simulink model "fuelCycle_w_trapping"  (R2023b)
settings: Solver=ode15s  StartTime=0.0  StopTime=sim_time  MinStep=1e-4  RelTol=1e-4
values from neighbouring files (symbols this model uses):
  AF = 0.90    (= 0.9)    [FC_scenario_inputData.m]    (also in inputData.m = 70)
  eta2 = 0.95    [FC_scenario_inputData.m]    (also in inputData.m)
  f51 = 0.33    [FC_scenario_inputData.m]    (also in inputData.m)
  f53 = 0.33    [FC_scenario_inputData.m]    (also in inputData.m)
  f54 = 1 - f51 - f53 - f56    (= 0.3399)    [FC_scenario_inputData.m]    (also in inputData.m)
  f96 = 0.1    [FC_scenario_inputData.m]    (also in inputData.m)
  f_dir = 0.7    [FC_scenario_inputData.m]    (also in inputData.m = 0.3)
  fp3 = 1e-4    (= 0.0001)    [FC_scenario_inputData.m]    (also in inputData.m; parametric_analysis_f_p_trap.m = f_p(i))
  fp4 = 1e-4    (= 0.0001)    [FC_scenario_inputData.m]    (also in inputData.m; parametric_analysis_f_p_trap.m = f_p(i))
  I_s_0 = 1.85    [fuelCycleSimulator.m]    (also in parametric_analysis_f_p_trap.m = 0.8; utilities.m = I_s_0 - abs(margin) + inventory_accuracy)
  lambda = 1.73e-9    (= 1.73e-09)    [FC_scenario_inputData.m]    (also in inputData.m)
  N_dot = 9.3e-7    (= 9.3e-07)    [FC_scenario_inputData.m]    (also in inputData.m)
  n_trap_structural = n_trap_vcrti    (= 0.0001)    [inputData_trapping.m]    (also in parametric_analysis_trapping.m = n_trap_array(j))
  n_trap_tungsten_intrinsic = 3.5e-4    (= 0.00035)    [inputData_trapping.m]
  T1 = 1/((1 + epsi)/tau1 + lambda)    [FC_scenario_inputData.m]    (also in inputData.m)
  T12 = 1/((1 + epsi)/tau12 + lambda)    [FC_scenario_inputData.m]    (also in inputData.m)
  T2 = 1/((1 + epsi)/tau2 + lambda)    [FC_scenario_inputData.m]    (also in inputData.m)
  T3 = 1/((1 + 0)/tau3 + lambda)    [FC_scenario_inputData.m]    (also in inputData.m)
  T4 = 1/((1 + 0)/tau4 + lambda)    [FC_scenario_inputData.m]    (also in inputData.m)
  T7 = 1/((1 + epsi)/tau7 + lambda)    [FC_scenario_inputData.m]    (also in inputData.m)
  T8 = 1/((1 + epsi)/tau8 + lambda)    [FC_scenario_inputData.m]    (also in inputData.m)
  T9 = 1/((1 + epsi)/tau9 + lambda)    [FC_scenario_inputData.m]    (also in inputData.m)
  T_replacement = 1.7*8760*3600    (= 53611200)    [inputData.m]
  tau1 = 1.25*3600    (= 4500)    [FC_scenario_inputData.m]    (also in inputData.m)
  tau12 = 100    [FC_scenario_inputData.m]    (also in inputData.m)
  tau2 = 1*24*3600    (= 86400)    [FC_scenario_inputData.m]    (also in inputData.m)
  tau3 = 1000    [FC_scenario_inputData.m]    (also in inputData.m)
  tau4 = 1000    [FC_scenario_inputData.m]    (also in inputData.m)
  tau5 = 1000    [FC_scenario_inputData.m]    (also in inputData.m)
  tau6 = 3600    [FC_scenario_inputData.m]    (also in inputData.m)
  tau7 = 600    [FC_scenario_inputData.m]    (also in inputData.m)
  tau8 = 0.1*3600    (= 360)    [FC_scenario_inputData.m]    (also in inputData.m = 3600)
  tau9 = 0.9*3600    (= 3240)    [FC_scenario_inputData.m]    (also in inputData.m = 10800)
  tau_detrap_structural = 1 / nu_detrap_structural* relaxation_coefficient    [inputData_trapping.m]
  TBE = 0.02    [FC_scenario_inputData.m]    (also in inputData.m; parametric_analysis_f_p_trap.m = TBE_array(j); parametric_analysis_trapping.m)
  TBR = 1.096    [fuelCycleSimulator.m]    (also in parametric_analysis_f_p_trap.m = 1.048; parametric_analysis_trapping.m = 1.06; utilities.m = TBR_start)
libraries: arc x5
settings Model: SimulationMode=accelerator  Creator=smesc  LastModifiedBy=smesc
settings SolverCC: InitialStep=1e-4  MaxConsecutiveMinStep=10  ShapePreserveControl=EnableAll  ZeroCrossAlgorithm=Adaptive
settings OptimizationCC: ReuseModelBlockBuffer=off
settings ModelReferenceCC: EnableRefExpFcnMdlSchedulingChecks=on

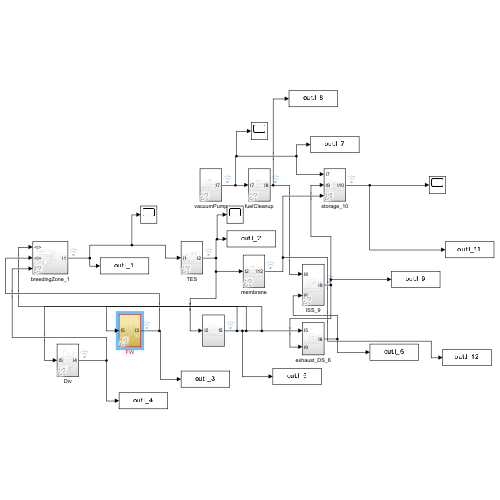
[thumbnail: Simulink's stored preview of the top-level diagram]
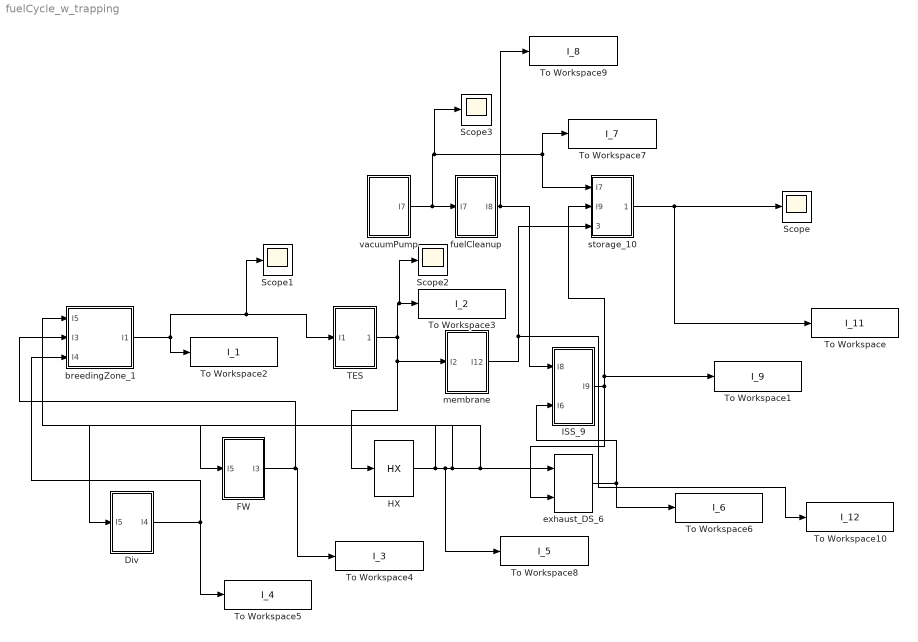
== system fuelCycle_w_trapping ==
  Div : Subsystem  AncestorBlock=arc/divertor_4
      settings: LibrarySourceBlock=arc/divertor_4
  FW : Subsystem  AncestorBlock=arc/FW_3
      settings: LibrarySourceBlock=arc/FW_3
  HX : arc/HX  Tag=HX  SystemSampleTime=-1  VariantActivationTime=update diagram  AllowFlexibleInterface=on  Latency=0  AutoFrameSizeCalculation=off
  ISS_9 : Subsystem  AncestorBlock=arc/ISS_9
      settings: LibrarySourceBlock=arc/ISS_9
  Scope{,1..3} (4 alike) : Scope
  TES : Subsystem  AncestorBlock=arc/TES_2
      settings: LibrarySourceBlock=arc/TES_2
  To Workspace : ToWorkspace  VariableName=I_11  SampleTime=-1
  To Workspace1 : ToWorkspace  VariableName=I_9  SampleTime=-1
  To Workspace10 : ToWorkspace  VariableName=I_12  SampleTime=-1
  To Workspace2 : ToWorkspace  VariableName=I_1  SampleTime=-1
  To Workspace3 : ToWorkspace  VariableName=I_2  SampleTime=-1
  To Workspace4 : ToWorkspace  VariableName=I_3  SampleTime=-1
  To Workspace5 : ToWorkspace  VariableName=I_4  SampleTime=-1
  To Workspace6 : ToWorkspace  VariableName=I_6  SampleTime=-1
  To Workspace7 : ToWorkspace  VariableName=I_7  SampleTime=-1
  To Workspace8 : ToWorkspace  VariableName=I_5  SampleTime=-1
  To Workspace9 : ToWorkspace  VariableName=I_8  SampleTime=-1
  breedingZone_1 : Subsystem  AncestorBlock=arc/breedingZone_1
      settings: LibrarySourceBlock=arc/breedingZone_1
  exhaust_DS_6 : arc/exhaust_DS  SystemSampleTime=-1  VariantActivationTime=update diagram  AllowFlexibleInterface=on  Latency=0  AutoFrameSizeCalculation=off
      link override Gain: Gain=f56/tau5
  fuelCleanup : Subsystem  AncestorBlock=arc/fuelCleanUp
  membrane : Subsystem  AncestorBlock=arc/fuelCleanUp_8
      settings: LibrarySourceBlock=arc/fuelCleanUp_8
  storage_10 : Subsystem  AncestorBlock=arc/storage_10
      settings: LibrarySourceBlock=arc/storage_10
  vacuumPump : Subsystem  AncestorBlock=arc/pump_7
      settings: LibrarySourceBlock=arc/pump_7
  wires:
  breedingZone_1/1(I1) -> Scope1/1, TES/1(I1), To Workspace2/1
  storage_10/1(I10) -> To Workspace/1, Scope/1
  FW/1(I3) -> breedingZone_1/2(I3), To Workspace4/1
  Div/1(I4) -> breedingZone_1/3(I4), To Workspace5/1
  membrane/1(I12) -> To Workspace10/1, storage_10/3(I12)
  fuelCleanup/1(I8) -> To Workspace9/1, ISS_9/1(I8)
  vacuumPump/1(I7) -> Scope3/1, To Workspace7/1, storage_10/1(I7), fuelCleanup/1(I7)
  exhaust_DS_6/1 -> ISS_9/2(I6), To Workspace6/1
  ISS_9/1(I9) -> exhaust_DS_6/2, storage_10/2(I9), To Workspace1/1
  HX/1 -> FW/1(I5), To Workspace8/1, Div/1(I5), exhaust_DS_6/1, breedingZone_1/1(I5)
  TES/1(Output) -> Scope2/1, To Workspace3/1, membrane/1(I2), HX/1

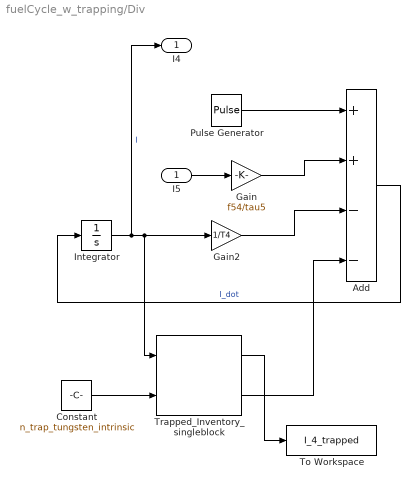
== system fuelCycle_w_trapping/Div ==
  I5 : Inport
  Add : Sum  Inputs=++--
  Constant : Constant  Value=n_trap_tungsten_intrinsic
  Gain : Gain  Gain=f54/tau5
  Gain2 : Gain  Gain=1/T4
  Integrator : Integrator
  Pulse Generator : DiscretePulseGenerator  PulseType=Time based  Amplitude=fp4*N_dot/TBE  Period=1800  PulseWidth=AF
  To Workspace : ToWorkspace  VariableName=I_4_trapped  SampleTime=-1
  Trapped_Inventory_singleblock : arc/Trapped_Inventory_singleblock  SystemSampleTime=-1  VariantActivationTime=update diagram  AllowFlexibleInterface=on  Latency=0  AutoFrameSizeCalculation=off
      link override Trap_detrap_ml2: tau_detrap=tau_detrap_tungsten(1)  n_solute=n_solute_tungsten  PM_host=PM_tungsten  M_host=PM_tungsten  tau_trap=tau_trap_tungsten
  I4 : Outport
  wires:
  Pulse Generator/1 -> Add/1
  Gain/1 -> Add/2
  Integrator/1 -> Trapped_Inventory_singleblock/1, Gain2/1, I4/1  "I"
  Add/1 -> Integrator/1  "I_dot"
  Gain2/1 -> Add/3
  I5/1 -> Gain/1
  Trapped_Inventory_singleblock/1 -> To Workspace/1
  Trapped_Inventory_singleblock/2 -> Add/4
  Constant/1 -> Trapped_Inventory_singleblock/2

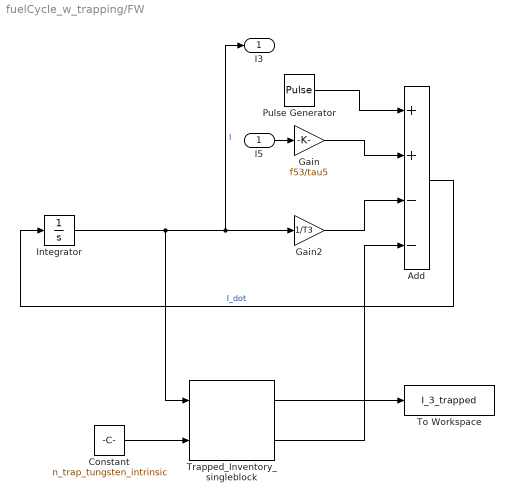
== system fuelCycle_w_trapping/FW ==
  I5 : Inport
  Add : Sum  Inputs=++--
  Constant : Constant  Value=n_trap_tungsten_intrinsic
  Gain : Gain  Gain=f53/tau5
  Gain2 : Gain  Gain=1/T3
  Integrator : Integrator
  Pulse Generator : DiscretePulseGenerator  PulseType=Time based  Amplitude=fp3*N_dot/TBE  Period=1800  PulseWidth=AF
  To Workspace : ToWorkspace  VariableName=I_3_trapped  SampleTime=-1
  Trapped_Inventory_singleblock : arc/Trapped_Inventory_singleblock  SystemSampleTime=-1  VariantActivationTime=update diagram  AllowFlexibleInterface=on  Latency=0  AutoFrameSizeCalculation=off
      link override Trap_detrap_ml2: tau_detrap=tau_detrap_tungsten(1)  n_solute=n_solute_tungsten  PM_host=PM_tungsten  M_host=M_tungsten  tau_trap=tau_trap_tungsten
  I3 : Outport
  wires:
  Gain2/1 -> Add/3
  Pulse Generator/1 -> Add/1
  Integrator/1 -> Gain2/1, I3/1, Trapped_Inventory_singleblock/1  "I"
  Add/1 -> Integrator/1  "I_dot"
  Gain/1 -> Add/2
  I5/1 -> Gain/1
  Trapped_Inventory_singleblock/2 -> Add/4
  Trapped_Inventory_singleblock/1 -> To Workspace/1
  Constant/1 -> Trapped_Inventory_singleblock/2

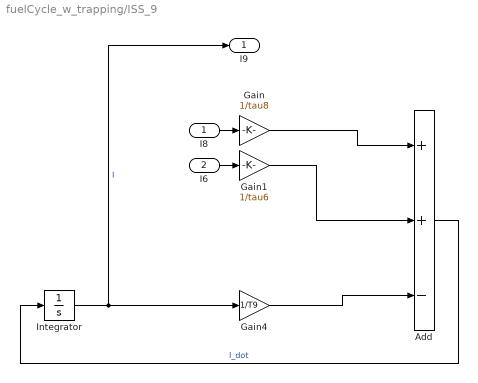
== system fuelCycle_w_trapping/ISS_9 ==
  I8 : Inport
  I6 : Inport  Port=2
  Add : Sum  Inputs=++-
  Gain : Gain  Gain=1/tau8
  Gain1 : Gain  Gain=1/tau6
  Gain4 : Gain  Gain=1/T9
  Integrator : Integrator
  I9 : Outport
  wires:
  I8/1 -> Gain/1
  Gain1/1 -> Add/2
  I6/1 -> Gain1/1
  Add/1 -> Integrator/1  "I_dot"
  Integrator/1 -> Gain4/1, I9/1  "I"
  Gain/1 -> Add/1
  Gain4/1 -> Add/3

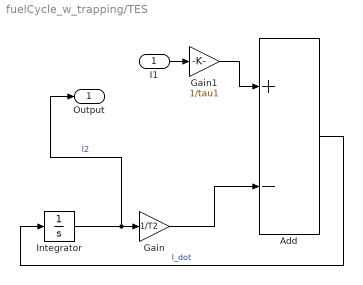
== system fuelCycle_w_trapping/TES ==
  I1 : Inport
  Add : Sum  Inputs=+-
  Gain : Gain  Gain=1/T2
  Gain1 : Gain  Gain=1/tau1
  Integrator : Integrator
  Output : Outport
  wires:
  Gain/1 -> Add/2
  I1/1 -> Gain1/1
  Gain1/1 -> Add/1
  Integrator/1 -> Gain/1, Output/1  "I2"
  Add/1 -> Integrator/1  "I_dot"

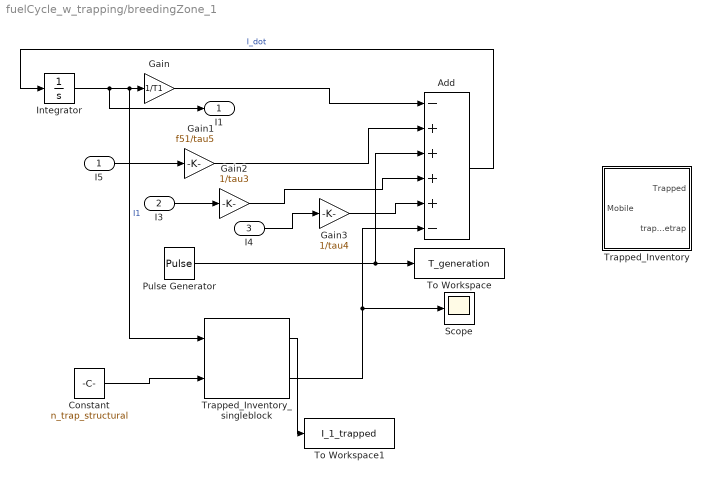
== system fuelCycle_w_trapping/breedingZone_1 ==
  I5 : Inport
  I3 : Inport  Port=2
  I4 : Inport  Port=3
  Add : Sum  Inputs=-++++-
  Constant : Constant  Value=n_trap_structural
  Gain : Gain  Gain=1/T1
  Gain1 : Gain  Gain=f51/tau5
  Gain2 : Gain  Gain=1/tau3
  Gain3 : Gain  Gain=1/tau4
  Integrator : Integrator
  Pulse Generator : DiscretePulseGenerator  PulseType=Time based  Amplitude=N_dot * TBR  Period=1800  PulseWidth=AF
  Scope : Scope
  To Workspace : ToWorkspace  VariableName=T_generation  SaveFormat=Timeseries  SampleTime=-1
  To Workspace1 : ToWorkspace  VariableName=I_1_trapped  SampleTime=-1
  Trapped_Inventory : Subsystem  AncestorBlock=arc/Trapped_Inventory
  Trapped_Inventory_singleblock : arc/Trapped_Inventory_singleblock  SystemSampleTime=-1  VariantActivationTime=update diagram  AllowFlexibleInterface=on  Latency=0  AutoFrameSizeCalculation=off
      link override Trap_detrap_ml2: tau_detrap=tau_detrap_structural  n_solute=n_solute_structural
  I1 : Outport
  wires:
  Add/1 -> Integrator/1  "I_dot"
  Gain1/1 -> Add/2
  Integrator/1 -> Trapped_Inventory_singleblock/1, Gain/1, I1/1  "I1"
  Gain/1 -> Add/1
  I5/1 -> Gain1/1
  Pulse Generator/1 -> Add/3, To Workspace/1
  I3/1 -> Gain2/1
  Gain2/1 -> Add/4
  I4/1 -> Gain3/1
  Gain3/1 -> Add/5
  Constant/1 -> Trapped_Inventory_singleblock/2
  Trapped_Inventory_singleblock/1 -> To Workspace1/1
  Trapped_Inventory_singleblock/2 -> Add/6, Scope/1

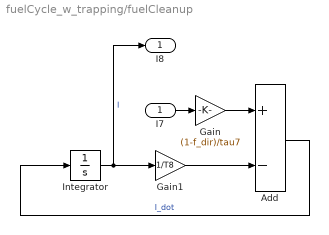
== system fuelCycle_w_trapping/fuelCleanup ==
  I7 : Inport
  Add : Sum  Inputs=+-
  Gain : Gain  Gain=(1-f_dir)/tau7
  Gain1 : Gain  Gain=1/T8
  Integrator : Integrator
  I8 : Outport
  wires:
  I7/1 -> Gain/1
  Gain1/1 -> Add/2
  Add/1 -> Integrator/1  "I_dot"
  Integrator/1 -> Gain1/1, I8/1  "I"
  Gain/1 -> Add/1

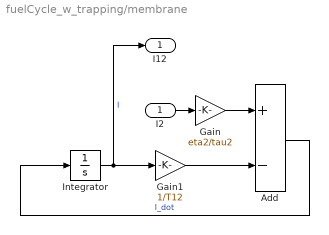
== system fuelCycle_w_trapping/membrane ==
  I2 : Inport
  Add : Sum  Inputs=+-
  Gain : Gain  Gain=eta2/tau2
  Gain1 : Gain  Gain=1/T12
  Integrator : Integrator
  I12 : Outport
  wires:
  I2/1 -> Gain/1
  Gain1/1 -> Add/2
  Add/1 -> Integrator/1  "I_dot"
  Integrator/1 -> Gain1/1, I12/1  "I"
  Gain/1 -> Add/1

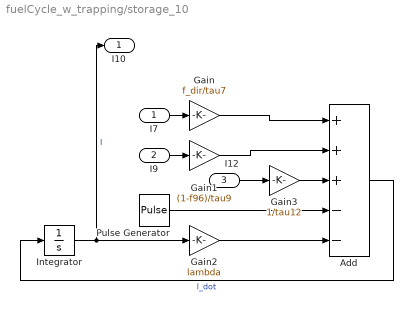
== system fuelCycle_w_trapping/storage_10 ==
  I7 : Inport
  I9 : Inport  Port=2
  I12 : Inport  Port=3
  Add : Sum  Inputs=+++--
  Gain : Gain  Gain=f_dir/tau7
  Gain1 : Gain  Gain=(1-f96)/tau9
  Gain2 : Gain  Gain=lambda
  Gain3 : Gain  Gain=1/tau12
  Integrator : Integrator  InitialCondition=I_s_0
  Pulse Generator : DiscretePulseGenerator  PulseType=Time based  Amplitude=N_dot/TBE  Period=1800  PulseWidth=AF
  I10 : Outport
  wires:
  Integrator/1 -> Gain2/1, I10/1  "I"
  I9/1 -> Gain1/1
  Gain2/1 -> Add/5
  I7/1 -> Gain/1
  Gain1/1 -> Add/2
  Gain/1 -> Add/1
  Pulse Generator/1 -> Add/4
  I12/1 -> Gain3/1
  Gain3/1 -> Add/3
  Add/1 -> Integrator/1  "I_dot"

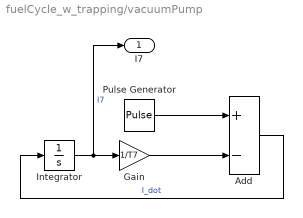
== system fuelCycle_w_trapping/vacuumPump ==
  Add : Sum  Inputs=+-
  Gain : Gain  Gain=1/T7
  Integrator : Integrator
  Pulse Generator : DiscretePulseGenerator  PulseType=Time based  Amplitude=(1-TBE-fp3-fp4)*N_dot/TBE  Period=1800  PulseWidth=AF
  I7 : Outport
  wires:
  Gain/1 -> Add/2
  Integrator/1 -> Gain/1, I7/1  "I7"
  Pulse Generator/1 -> Add/1
  Add/1 -> Integrator/1  "I_dot"

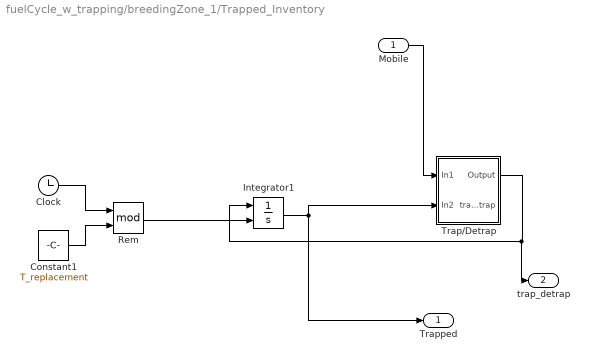
== system fuelCycle_w_trapping/breedingZone_1/Trapped_Inventory ==
  Mobile : Inport
  Clock : Clock
  Constant1 : Constant  Value=T_replacement
  Integrator1 : Integrator  ExternalReset=falling
  Rem : Math  Operator=mod
  Trap/Detrap : Subsystem
  Trapped : Outport
  trap_detrap : Outport  Port=2
  wires:
  Trap/Detrap/1(Output) -> trap_detrap/1, Integrator1/1
  Mobile/1 -> Trap/Detrap/1(In1)
  Integrator1/1 -> Trap/Detrap/2(In2), Trapped/1
  Clock/1 -> Rem/1
  Rem/1 -> Integrator1/2
  Constant1/1 -> Rem/2

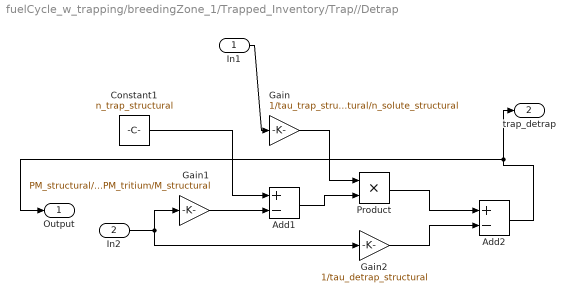
== system fuelCycle_w_trapping/breedingZone_1/Trapped_Inventory/Trap//Detrap ==
  In1 : Inport
  In2 : Inport  Port=2
  Add1 : Sum  Inputs=+-
  Add2 : Sum  Inputs=+-
  Constant1 : Constant  Value=n_trap_structural
  Gain : Gain  Gain=1/tau_trap_structural/n_solute_structural
  Gain1 : Gain  Gain=PM_structural/PM_tritium/M_structural
  Gain2 : Gain  Gain=1/tau_detrap_structural
  Product : Product
  Output : Outport
  trap_detrap : Outport  Port=2
  wires:
  In2/1 -> Gain1/1, Gain2/1
  Gain1/1 -> Add1/2
  Add1/1 -> Product/2
  Gain2/1 -> Add2/2
  Gain/1 -> Product/1
  In1/1 -> Gain/1
  Add2/1 -> trap_detrap/1, Output/1
  Product/1 -> Add2/1
  Constant1/1 -> Add1/1
